simulink model "adip_pcont_least_square_sim"  (R2013a)
settings: Solver=ode4  StartTime=0.0  StopTime=8  FixedStep=0.001  RelTol=1e-3
values from neighbouring files (symbols this model uses):
  a1 = 2*zeta*omega_n    [p1c332_adip_id_arm.m]    (also in p1c332_adip_id_least_square.m = p1(1))
  alpha2 = p2(1)    [p1c332_adip_id_least_square.m]
  alpha3 = m2*L1*l2    (= 0.00424944)    [p1c332_adip_id_least_square.m]
  alpha5 = m2*l2*g    (= 0.1836432)    [p1c332_adip_id_least_square.m]
  b1 = omega_n^2/kP    [p1c332_adip_id_arm.m]    (also in p1c332_adip_id_least_square.m = p1(2))
  kP = 10    [p1c321_cdip_id_cart.m]    (also in p1c322_cdip_id_least_square.m; p1c322_cdip_plot_MN.m; p1c332_adip_id_arm.m = 3; p1c332_adip_id_least_square.m = 3)
  mu2 = p2(2)    [p1c332_adip_id_least_square.m]    (also in p1c332_adip_id_pend.m = 2*zeta*omega_n*(J2 + m2*l2^2))
settings Model: Creator=kawata  LastModifiedBy=kawata

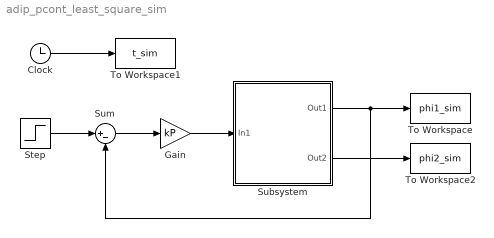
== system adip_pcont_least_square_sim ==
  Clock : Clock
  Gain : Gain  Gain=kP  SaturateOnIntegerOverflow=on  OutDataTypeStr=Inherit: Same as input  ParamDataTypeStr=Inherit: Same as input
  Step : Step  Time=0  SampleTime=0
  Subsystem : Subsystem
  Sum : Sum  Inputs=|+-  SaturateOnIntegerOverflow=on  InputSameDT=on  OutDataTypeStr=Inherit: Same as first input
  To Workspace : ToWorkspace  VariableName=phi1_sim  SampleTime=-1
  To Workspace1 : ToWorkspace  VariableName=t_sim  SampleTime=-1
  To Workspace2 : ToWorkspace  VariableName=phi2_sim  SampleTime=-1
  wires:
  Subsystem/1(Out1) -> Sum/2, To Workspace/1
  Step/1 -> Sum/1
  Sum/1 -> Gain/1
  Gain/1 -> Subsystem/1(In1)
  Subsystem/2(Out2) -> To Workspace2/1
  Clock/1 -> To Workspace1/1

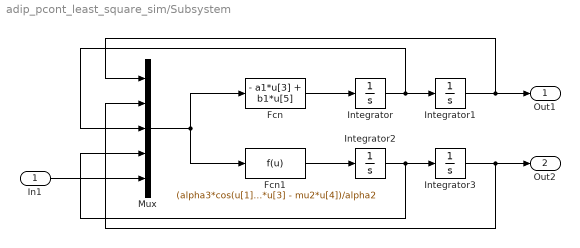
== system adip_pcont_least_square_sim/Subsystem ==
  In1 : Inport
  Fcn : Fcn  Expr=- a1*u[3] + b1*u[5]
  Fcn1 : Fcn  Expr=(alpha3*cos(u[1] - u[2])*(- a1*u[3] + b1*u[5]) - alpha3*u[3]^2*sin(u[1] - u[2]) - alpha5*sin(u[2]) + mu2*u[3] - mu2*u[4])/alpha2
  Integrator{,1..3} (4 alike) : Integrator
  Mux : Mux  Inputs=5
  Out1 : Outport
  Out2 : Outport  Port=2
  wires:
  Integrator1/1 -> Mux/1, Out1/1
  In1/1 -> Mux/5
  Integrator3/1 -> Out2/1, Mux/2
  Mux/1 -> Fcn1/1, Fcn/1
  Fcn1/1 -> Integrator2/1
  Integrator2/1 -> Mux/4, Integrator3/1
  Integrator/1 -> Mux/3, Integrator1/1
  Fcn/1 -> Integrator/1
